simulink model "subsys"  (Simulink 6.6)
settings: Solver=ode45  StartTime=0.0  StopTime=2.515  RelTol=1e-3
libraries: simulink x1
settings Model: Creator=student  LastModifiedBy=student

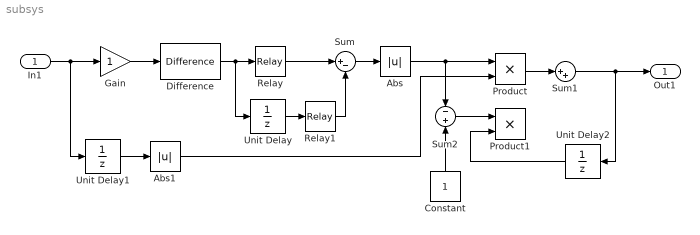
== system subsys ==
  In1 : Inport
  Abs : Abs
  Abs1 : Abs
  Constant : Constant  Orientation=up
  Difference : simulink/Discrete/Difference  SystemSampleTime=-1  ICPrevInput=0.0  OutDataType=sfix(16)  OutScaling=2^-10  DoSatur=off
  Gain : Gain
  Product : Product  RndMeth=Zero
  Product1 : Product  RndMeth=Zero
  Relay : Relay
  Relay1 : Relay
  Sum : Sum  Inputs=|+-
  Sum1 : Sum  Inputs=|++
  Sum2 : Sum  Inputs=-|+
  Unit Delay : UnitDelay
  Unit Delay1 : UnitDelay
  Unit Delay2 : UnitDelay  Orientation=left
  Out1 : Outport
  wires:
  In1/1 -> Gain/1, Unit Delay1/1
  Gain/1 -> Difference/1
  Unit Delay/1 -> Relay1/1
  Difference/1 -> Relay/1, Unit Delay/1
  Relay/1 -> Sum/1
  Relay1/1 -> Sum/2
  Sum/1 -> Abs/1
  Abs/1 -> Product/1, Sum2/1
  Unit Delay1/1 -> Abs1/1
  Product/1 -> Sum1/1
  Abs1/1 -> Product/2
  Constant/1 -> Sum2/2
  Sum2/1 -> Product1/1
  Unit Delay2/1 -> Product1/2
  Sum1/1 -> Out1/1, Unit Delay2/1
